simulink model "problem4"  (R2020b)
settings: Solver=VariableStepAuto  StartTime=0.0  StopTime=10.0  MaxStep=0.01  RelTol=1e-3
settings Model: Creator=lalit  LastModifiedBy=lalit

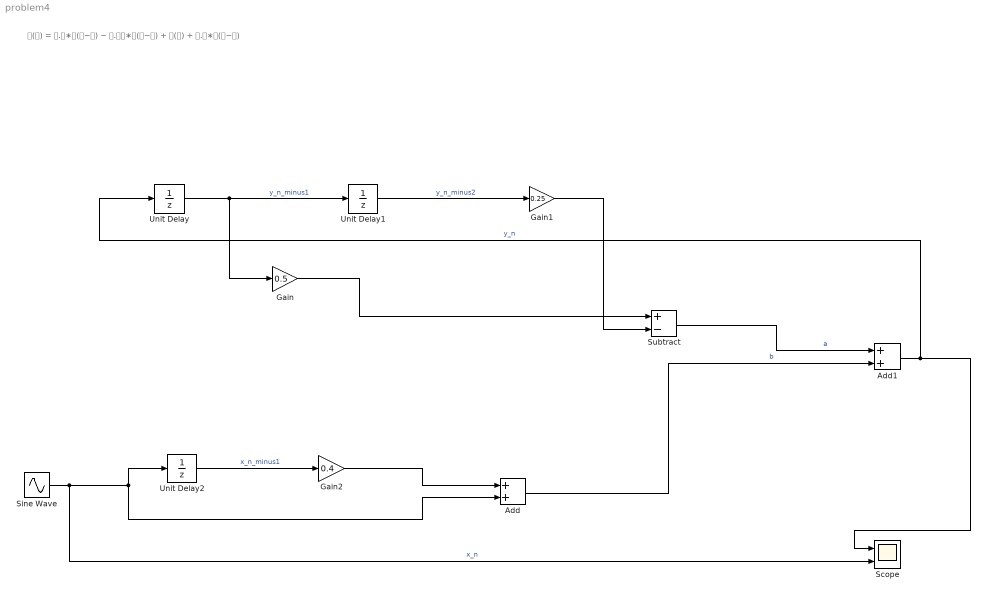
== system problem4 ==
  note: 𝐲(𝐧) = 𝟎.𝟓∗𝐲(𝐧−𝟏) − 𝟎.𝟐𝟓∗𝐲(𝐧−𝟐) + 𝐱(𝐧) + 𝟎.𝟒∗𝐱(𝐧−𝟏)
  Add : Sum
  Add1 : Sum
  Gain : Gain  Gain=0.5
  Gain1 : Gain  Gain=0.25
  Gain2 : Gain  Gain=0.4
  Scope : Scope  NumInputPorts=2
  Sine Wave : Sin  Amplitude=5  Frequency=20  SampleTime=0
  Subtract : Sum  Inputs=+-
  Unit Delay : UnitDelay  SampleTime=-1  HasFrameUpgradeWarning=on
  Unit Delay1 : UnitDelay  SampleTime=-1  HasFrameUpgradeWarning=on
  Unit Delay2 : UnitDelay  SampleTime=-1  HasFrameUpgradeWarning=on
  wires:
  Add1/1 -> Unit Delay/1, Scope/1  "y_n"
  Unit Delay/1 -> Gain/1, Unit Delay1/1  "y_n_minus1"
  Unit Delay1/1 -> Gain1/1  "y_n_minus2"
  Unit Delay2/1 -> Gain2/1  "x_n_minus1"
  Gain/1 -> Subtract/1
  Gain1/1 -> Subtract/2
  Subtract/1 -> Add1/1  "a"
  Gain2/1 -> Add/1
  Add/1 -> Add1/2  "b"
  Sine Wave/1 -> Scope/2, Add/2, Unit Delay2/1  "x_n"
